simulink model "armed_trigger_blk"  (R2019a)
settings: Solver=VariableStepAuto  StartTime=0.0  StopTime=10.0  RelTol=1e-3
libraries: xbsIndex_r4 x1
settings Model: Creator=mybur  LastModifiedBy=mybur

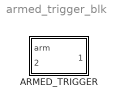
== system armed_trigger_blk ==
  ARMED_TRIGGER : Subsystem
      mask DialogControl DescTextVar Prompt: Makes a boolean trigger signal armable.

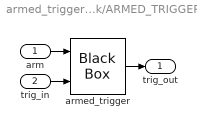
== system armed_trigger_blk/ARMED_TRIGGER ==
  arm : Inport
  trig_in : Inport  Port=2
  armed_trigger : xbsIndex_r4/Black Box  init_code=armed_trigger_config  sim_method=ISE Simulator  verbose=off  block_type=blackbox2
  trig_out : Outport
  wires:
  arm/1 -> armed_trigger/1
  trig_in/1 -> armed_trigger/2
  armed_trigger/1 -> trig_out/1
